simulink model "mpptprabanshv2"  (R2019a)
settings: Solver=ode23t  StartTime=0.0  StopTime=10  RelTol=1e-3
undefined symbols (not defined in the file): Ion, Lithium
libraries: powerlib x20, electricdrivelib x2, re_lib x1, powerlib_meascontrol x1
settings Model: Creator=dell  LastModifiedBy=Dell
settings SolverCC: AlgebraicLoopSolver=LineSearch

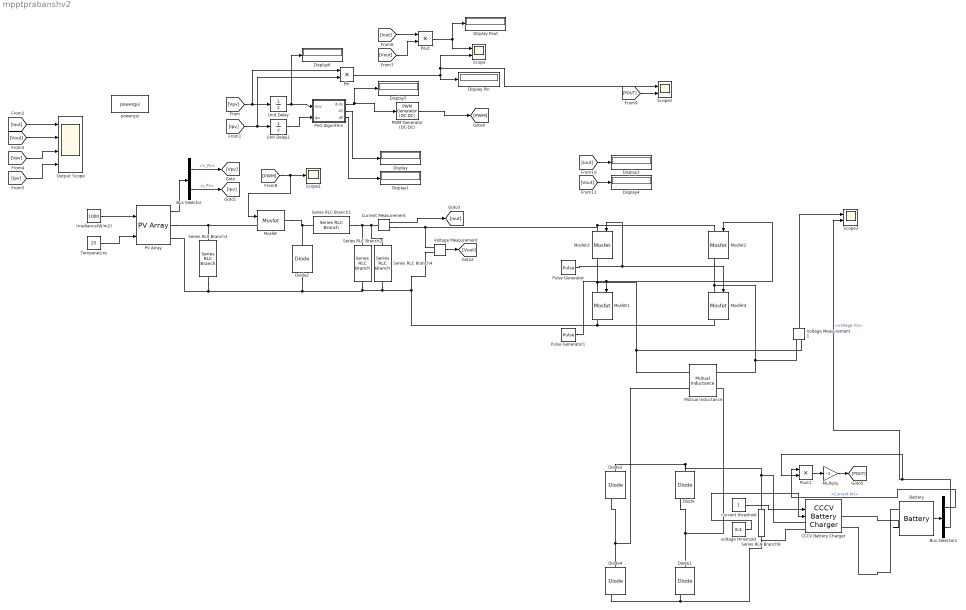
== system mpptprabanshv2 ==
  Battery : electricdrivelib/Extra Sources/Battery  BatType=Lithium-Ion  ShowTempParam=off  ThermalPreset=no  ShowAgeParam=off  NomV=8.4  NomQ=5.4  SOC=20  Batt_Tr=30  PresetModel=on  MaxQ=5.4  MinV=6.3  FullV=9.7775  Dis_rate=2.3478  R=0.015556  Normal_OP=4.8835  expZone="[9.0752      0.2653]"  current=[6.5 13 32.5]  Units=Time  Tci=20  NomT=20  T2=-30  MaxQ2=4.8  FullV2=7.1  Normal_OP2=5.655  expZone2="[6.58           1]"  Rca=0.6  ti=2000  Dp=0  Neq0=0  Tsim=1e6  Ta1=25  Qeol=5.4*0.9  Reol=0.013333*1.2  Char_age=[2.3478, 3]  Dis_age=[2.3478, 10]  N1=1500  N2=10500  N3=1000  N4=1400  Ta2=45  N5=950
      settings: SourceProductName=Simscape Electrical
  Bus Selector : BusSelector  OutputSignals=V_PV,I_PV
  Bus Selector1 : BusSelector  OutputSignals=Current (A),Voltage (V)
  CCCV Battery Charger : electricdrivelib/Extra Sources/CCCV Battery Charger  Preset=Custom specifications  P_nom=1500  s_type=DC  n_connect=off  eff_volt=20  in_freq=60  in_I_ripple=10  in_I_freq=1000  EFF_en=on  EFF_val=[0.627 0.803 0.855 0.871 0.872 0.864]  EFF_fu=[0.063 0.177 0.293 0.483 0.674 0.914]  THD_en=on  I_THD_val=[0.327 0.394 0.394 0.351 0.289 0.265]  I_THD_fu=[0.056 0.136 0.194 0.303 0.555 0.916]  H_DIST_rt=[0.199 1.297 0.328 0.029 0.416 0.200]  H_DIST_fr=[3 5 7 9 11 13]  PF_en=on  PF_val=[0.316 0.532 0.662 0.731 0.780 0.792]  PF_fu=[0.067 0.230 0.445 0.625 0.794 0.919]  Out_mode=Constant Current - Constant Voltage (CCCV)  DynInT=on  I_cst=2  V_cst=8.4  ABS_en=off  V_abs=142  ABS_end=Time based  ABS_time=3600  ABS_i=40  ripple=0.5  swF=1000  overshoot=1  stable_t=5  VoltComp=on  V_comp=-0.18  nom_temp=27
      settings: SourceProductName=Simscape Electrical  SourceProductBaseCode=PS
  Current Measurement : powerlib/Measurements/Current Measurement  PhasorSimulation=off  OutputType=Complex  PSBequivalent=0
      settings: SourceProductName=Simscape Electrical
  Diode{,1,3..4} (4 alike) : powerlib/Power Electronics/Diode  Ron=0.001  Lon=0  Vf=0.7  IC=0  UseSnubber=0  Rs=500  Cs=250e-9  Measurements=on
      settings: SourceProductName=Simscape Electrical
  Diode2 : powerlib/Power Electronics/Diode  Ron=0.001  Lon=0  Vf=0.8  IC=0  UseSnubber=0  Rs=inf  Cs=250e-9  Measurements=off
      settings: SourceProductName=Simscape Electrical
  Display{,1,3..6} (6 alike) : Display
  Display Pin : Display
  Display Pout : Display
  Irradiance(W/m2) : Constant  Value=1000
  Mosfet : powerlib/Power Electronics/Mosfet  Ron=0.1  Lon=0  Rd=0.01  Vfd=0  IC=0  Rs=1e5  Cs=inf  Measurements=off
      settings: SourceProductName=Simscape Electrical
  Mosfet{1..4} (4 alike) : powerlib/Power Electronics/Mosfet  Ron=0.1  Lon=0  Rd=0.01  Vfd=0  IC=0  Rs=1e5  Cs=inf  Measurements=on
      settings: SourceProductName=Simscape Electrical
  Multiply : Gain  Gain=-1
  Mutual Inductance : powerlib/Elements/Mutual Inductance  LConnTagsString=a|b  RConnTagsString=A|B  TypeOfMutual=Two or three windings with equal mutual terms  NumberOfWindings=3  SelfImpedance1=[1.1 1.1e-03]  SelfImpedance2=[ 1.1 1.1e-03]  ThreeWindings=off  SelfImpedance3=[ 1.1 1.1e-03]  MutualImpedance=[1.0 1.0e-03]  InductanceMatrix="[1.0 0.9  0.9 ;  0.9 1.0  0.9;  0.9 0.9 1.0 ] * 1e-3"  ResistanceMatrix="[1.0 0.9  0.9 ;  0.9 1.0  0.9;  0.9 0.9 1.0 ]"  Measurements=None
      settings: AttributesFormatString=\n  SourceProductName=Simscape Electrical  SourceProductBaseCode=PS
  Output Scope : Scope  NumInputPorts=4
  PV Array : re_lib/Solar/PV Array  Npar=1  Nser=1  PlotType=array @ 25 deg.C & specified irradiances  S_vec=1000  Temp_C_vec="[ 45 25  ]"  ModuleName=User-defined  PlotWhenSelected=off  Pm=10.01  Ncell=36  Voc=22.50  Isc=0.55  Vm=19.25  Im=0.52  beta_Voc_pc=-0.36099  alpha_Isc_pc=0.102  beta_Voc=-0.081223  alpha_Isc=0.000561  IL=0.55009  I0=2.0509e-11  nI=1.0135  Rsh=4393.6866  Rs=0.73892  BAL=on  Tc=1e-6  Tfilter=5e-5
      settings: SourceProductName=Simscape Electrical
  PWM Generator (DC-DC) : powerlib_meascontrol/Pulse & Signal Generators/PWM Generator (DC-DC)  Fsw=5000  Ts=0
      settings: SourceProductName=Simscape Electrical
  Pin : Product
  PnO Algorithm : MATLAB Function  TreatAsAtomicUnit=on
  Pout : Product
  Pout1 : Product
  Pulse Generator : DiscretePulseGenerator  PulseType=Time based  Amplitude=5  Period=2e-4  PulseWidth=50
  Pulse Generator1 : DiscretePulseGenerator  PulseType=Time based  Amplitude=5  Period=2e-4  PulseWidth=50  PhaseDelay=1e-4
  Scope : Scope  NumInputPorts=2
  Scope1 : Scope
  Scope2 : Scope  NumInputPorts=2
  Scope3 : Scope  NumInputPorts=2
  Series RLC Branch1 : powerlib/Elements/Series RLC Branch  LConnTagsString=__new0  RConnTagsString=__new0  BranchType=L  Resistance=1  Inductance=0.783e-3  SetiL0=off  InitialCurrent=0  Capacitance=10e-6  Setx0=off  InitialVoltage=0  Measurements=None
      settings: SourceProductName=Simscape Electrical
  Series RLC Branch2 : powerlib/Elements/Series RLC Branch  LConnTagsString=__new0  RConnTagsString=__new0  BranchType=C  Resistance=1  Inductance=1e-3  SetiL0=off  InitialCurrent=0  Capacitance=364e-6  Setx0=off  InitialVoltage=0  Measurements=None
      settings: SourceProductName=Simscape Electrical
  Series RLC Branch3 : powerlib/Elements/Series RLC Branch  LConnTagsString=__new0  RConnTagsString=__new0  BranchType=RC  Resistance=1e-3  Inductance=1e-3  SetiL0=off  InitialCurrent=0  Capacitance=1000e-6  Setx0=off  InitialVoltage=0  Measurements=None
      settings: SourceProductName=Simscape Electrical
  Series RLC Branch4 : powerlib/Elements/Series RLC Branch  LConnTagsString=__new0  RConnTagsString=__new0  BranchType=R  Resistance=10  Inductance=1e-3  SetiL0=off  InitialCurrent=0  Capacitance=364e-6  Setx0=off  InitialVoltage=0  Measurements=None
      settings: SourceProductName=Simscape Electrical
  Series RLC Branch6 : powerlib/Elements/Series RLC Branch  LConnTagsString=__new0  RConnTagsString=__new0  BranchType=C  Resistance=1000  Inductance=1e-3  SetiL0=off  InitialCurrent=0  Capacitance=1000e-6  Setx0=off  InitialVoltage=0  Measurements=None
      settings: SourceProductName=Simscape Electrical
  Temperature : Constant  Value=25
  Unit Delay : UnitDelay  SampleTime=1e-4  HasFrameUpgradeWarning=on
  Unit Delay1 : UnitDelay  SampleTime=1e-4  HasFrameUpgradeWarning=on
  Voltage Measurement : powerlib/Measurements/Voltage Measurement  PhasorSimulation=off  OutputType=Complex  PSBequivalent=0
      settings: SourceProductName=Simscape Electrical
  Voltage Measurement1 : powerlib/Measurements/Voltage Measurement  PhasorSimulation=off  OutputType=Complex  PSBequivalent=0
      settings: SourceProductName=Simscape Electrical
  current threshold : Constant
  powergui : powerlib/powergui  Priority=1  SimulationMode=Discrete  SampleTime=10e-6  frequency=60  Iterations=50  frequencyindice=0  Pbase=100e6  ErrMax=1e-4  UnitsV=kV  UnitsW=MW  buscounter=0  FunctionMessages=off  echomessages=off  EnableUseOfTLC=off  CurrentSourceSwitches=off  DisableSnubberDevices=off  DisableRonSwitches=off  DisableVfSwitches=off  DisplayEquations=off  AutomaticDiscreteSolvers=off  SolverType=Tustin/Backward Euler (TBE)  Interpol=off  ExternalGateDelay=off  methode=off  Ts=100  x0status=blocks  SPID=on  SwTol=0  HookPort=off  NonlinearTolerance=0  nMaxIteration=15  ContinueOnMaxIteration=off  RestoreLinks=warning  ResistiveCurrentMeasurement=off  Frange=[0:2:500]  Ylog=off  Xlog=on  ShowGrid=off  save=off  variable=ZData  structure=0  ZoomFFT=off  StartTime=0.0  cycles=1  DisplayStyle=1  fundamental=60  FreqAxis=off  MaxFrequency=1000  frequencyindicesteady=1  RmsSteady=1  display=off
      settings: SourceProductName=Simscape Electrical
  voltage threshold : Constant  Value=8.4
  wires:
  Irradiance(W/m2)/1 -> PV Array/1
  Temperature/1 -> PV Array/2
  PV Array/1 -> Bus Selector/1
  Bus Selector/2 -> [Ipv]  "<I_PV>"
  Bus Selector/1 -> [Vpv]  "<V_PV>"
  [Iout] -> Output Scope/1
  [Vout] -> Output Scope/2
  [Vpv] -> Output Scope/3
  [Ipv] -> Output Scope/4
  [Iout] -> Pout/1
  [Vout] -> Pout/2
  [Vpv] -> Pin/1, Unit Delay/1
  Unit Delay/1 -> Display6/1, PnO Algorithm/1(Vpv)
  [Ipv] -> Pin/2, Unit Delay1/1
  Unit Delay1/1 -> PnO Algorithm/2(Ipv)
  Pout/1 -> Display Pout/1, Scope/1
  Pin/1 -> Scope/2, Scope2/1, Display Pin/1
  PnO Algorithm/1(duty) -> PWM Generator (DC-DC)/1, Display5/1
  [PWM] -> Scope1/1, Mosfet/1
  PnO Algorithm/2(dV) -> Display/1
  PnO Algorithm/3(dP) -> Display1/1
  [Iout] -> Display3/1
  [Vout] -> Display4/1
  PWM Generator (DC-DC)/1 -> [PWM]
  Voltage Measurement/1 -> [Vout]
  Current Measurement/1 -> [Iout]
  Pulse Generator/1 -> Mosfet3/1, Mosfet4/1
  Voltage Measurement1/1 -> Scope3/1
  Pulse Generator1/1 -> Mosfet2/1, Mosfet1/1
  [POUT] -> Scope2/2
  Battery/1 -> Bus Selector1/1
  Bus Selector1/1 -> Pout1/1  "<Current (A)>"
  Bus Selector1/2 -> Pout1/2, Scope3/2  "<Voltage (V)>"
  current threshold/1 -> CCCV Battery Charger/2
  voltage threshold/1 -> CCCV Battery Charger/3
  Pout1/1 -> Multiply/1
  Multiply/1 -> [POUT]
  connections:
  Series RLC Branch1/LConn1 -- Series RLC Branch4/LConn1 -- Current Measurement/LConn1 -- Series RLC Branch2/LConn1
  PV Array/RConn1 -- Mosfet/LConn1 -- Series RLC Branch3/LConn1
  Mosfet/RConn1 -- Diode2/RConn1 -- Series RLC Branch1/RConn1
  Mosfet4/LConn1 -- Mosfet2/RConn1 -- Mutual Inductance/RConn1 -- Voltage Measurement1/LConn1
  Mosfet1/LConn1 -- Mutual Inductance/LConn1 -- Voltage Measurement1/LConn2 -- Mosfet3/RConn1
  Diode3/LConn1 -- CCCV Battery Charger/LConn1 -- Series RLC Branch6/LConn1 -- Diode/LConn1
  Diode4/LConn1 -- Mutual Inductance/LConn2 -- Diode3/RConn1
  Diode1/RConn1 -- CCCV Battery Charger/LConn2 -- Series RLC Branch6/RConn1 -- Diode4/RConn1
  Mutual Inductance/RConn2 -- Diode1/LConn1 -- Diode/RConn1
  Current Measurement/RConn1 -- Mosfet2/LConn1 -- Mosfet3/LConn1 -- Voltage Measurement/LConn1
  Series RLC Branch2/RConn1 -- Series RLC Branch4/RConn1 -- Voltage Measurement/LConn2 -- Mosfet4/RConn1 -- Mosfet1/RConn1 -- Diode2/LConn1 -- Series RLC Branch3/RConn1 -- PV Array/RConn2
  Battery/LConn1 -- CCCV Battery Charger/RConn1
  Battery/LConn2 -- CCCV Battery Charger/RConn2

== matlab function mpptprabanshv2/PnO Algorithm ==
  settings: updateMethod=DISCRETE
  data: Vpv input; duty output; Ipv input; dV output; dP output
function [duty,dV,dP] = PnO(Vpv, Ipv)
 
dutymax = 0.95;
dutymin = 0;
dutyinit = 0.95;
deltaduty = 0.001;
persistent Vold Pold dutyold;

dataType = 'double';

if isempty(Vold)
    Vold = 16.92;
    Pold = 9.2;
    dutyold = dutyinit;
end

Ppv = Vpv*Ipv;
dV = Vpv - Vold;
dP = Ppv - Pold;

if dP ~= 0
    if dP<0
        if dV<0
            duty = dutyold - deltaduty;
        else
            duty = dutyold + deltaduty;
        end
    else
        if dV<0
            duty = dutyold + deltaduty;
        else
            duty = dutyold - deltaduty;
        end
    end
else duty = dutyold;
end

%if duty >=dutymax | duty<= dutymin
%    duty = dutyold;
%end

dutyold = duty;
Vold = Vpv
Pold = Ppv;
